simulink model "Examen3s"  (R2015b)
settings: Solver=VariableStepAuto  StartTime=0.0  StopTime=3  RelTol=1e-3
libraries: fl_lib x19, nesl_utility x8
settings Model: Creator=xmax1946  LastModifiedBy=xmax1946

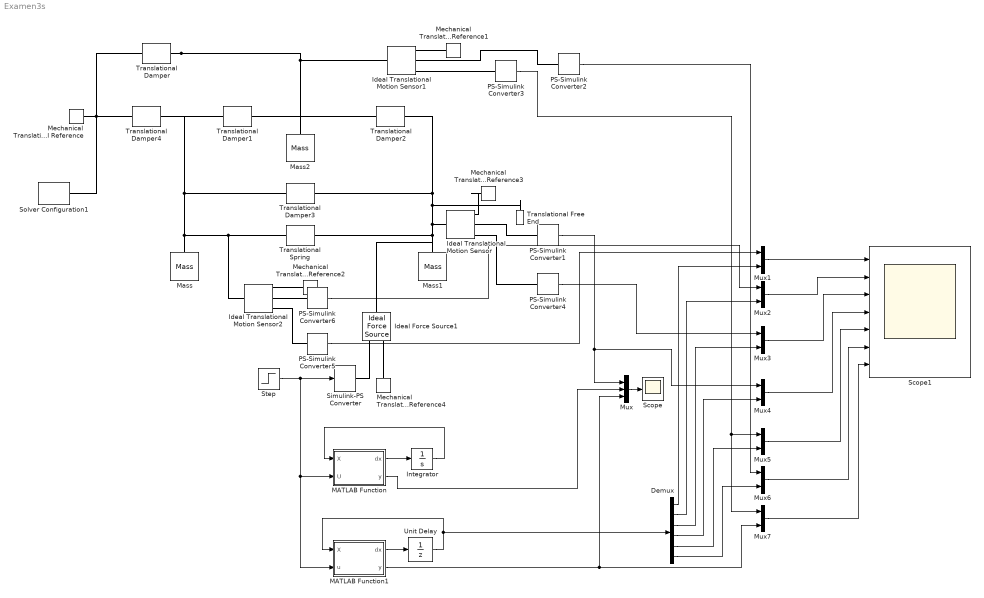
== system Examen3s ==
  Demux : Demux  Outputs=6
  Ideal Force Source1 : fl_lib/Mechanical/Mechanical Sources/Ideal Force Source
  Ideal Translational Motion Sensor : fl_lib/Mechanical/Mechanical Sensors/Ideal Translational Motion Sensor  offset=0 m
  Ideal Translational Motion Sensor1 : fl_lib/Mechanical/Mechanical Sensors/Ideal Translational Motion Sensor  offset=0 m
  Ideal Translational Motion Sensor2 : fl_lib/Mechanical/Mechanical Sensors/Ideal Translational Motion Sensor  offset=0 m
  Integrator : Integrator  InitialCondition=[0;0;0;0;0;0]
  MATLAB Function : MATLAB Function  TreatAsAtomicUnit=on
  MATLAB Function1 : MATLAB Function  TreatAsAtomicUnit=on
  Mass : fl_lib/Mechanical/Translational Elements/Mass  mass=2 kg  v_specify=off  v_priority=None  v=0 m/s  f_specify=off  f_priority=None  f=0 N
  Mass1 : fl_lib/Mechanical/Translational Elements/Mass  mass=1 kg  v_specify=off  v_priority=None  v=0 m/s  f_specify=off  f_priority=None  f=0 N
  Mass2 : fl_lib/Mechanical/Translational Elements/Mass  mass=1 kg  v_specify=off  v_priority=None  v=0 m/s  f_specify=off  f_priority=None  f=0 N
  Mechanical Translational Reference{,1..4} (5 alike) : fl_lib/Mechanical/Translational Elements/Mechanical Translational Reference
  Mux : Mux  Inputs=3
  Mux{1..7} (7 alike) : Mux  Inputs=2
  PS-Simulink Converter{1..6} (6 alike) : nesl_utility/PS-Simulink Converter  PhysicalDomain=network_engine_domain  SubClassName=ps_output  LeftPortType=input  RightPortType=output  PseudoPeriodic=off  Frequencies=[]  Unit=1  AffineConversion=off
  Scope : Scope
  Scope1 : Scope  NumInputPorts=7
  Simulink-PS Converter : nesl_utility/Simulink-PS Converter  PhysicalDomain=network_engine_domain  SubClassName=ps_input  LeftPortType=input  RightPortType=output  PseudoPeriodic=off  Frequencies=[]  NoiseDistribution=none  NoiseParameters=[]  Unit=1  AffineConversion=off  InputFiltering=off  SimscapeFilterOrder=1  InputFilterTimeConstant=0.001  UdotUserProvided=1
  Solver Configuration1 : nesl_utility/Solver Configuration  PhysicalDomain=network_engine_domain  SubClassName=solver  LeftPortType=input  RightPortType=generic  Accelerate=off  Tones=[]  Harmonics=[]  SimulateNoise=off  Profile=off  UseLocalSampling=off  EnableSwitchedLinearOptims=on  FrequencyDomain=off  UseCCode=off  RelTol=0.001  AbsTol=1e-06  MinStep=1e-09  ToWorkspace=off  RevertToSquareIcSolve=off  NumHomotopyIterations=100  PhasorMode=off  PhasorModeNumHarmonics=1  DoDC=off  ResidualTolerance=1e-09  UseLocalSolver=off  LocalSolverChoice=NE_BACKWARD_EULER_ADVANCER  LocalSolverSampleTime=0.001  DoFixedCost=off  MaxNonlinIter=3  MaxModeIter=2  LinearAlgebra=Sparse  DelaysMemoryBudget=1024  AutomaticFiltering=on  FilteringTimeConstant=0.001
  Step : Step  Time=0  SampleTime=0
  Translational Damper{,1..4} (5 alike) : fl_lib/Mechanical/Translational Elements/Translational Damper  D=1 N/(m/s)  v_specify=off  v_priority=None  v=0 m/s  f_specify=off  f_priority=None  f=0 N
  Translational Free End : fl_lib/Mechanical/Translational Elements/Translational Free End  v_specify=off  v_priority=None  v=0 m/s
  Translational Spring : fl_lib/Mechanical/Translational Elements/Translational Spring  spr_rate=2 N/m  v_specify=off  v_priority=None  v=0 m/s  f_specify=off  f_priority=None  f=0 N  x_specify=off  x_priority=None  x=0 m
  Unit Delay : UnitDelay  InitialCondition=[0;0;0;0;0;0]  SampleTime=.1
  wires:
  Step/1 -> MATLAB Function1/2(u), MATLAB Function/2(U), Simulink-PS Converter/1
  MATLAB Function/1(dx) -> Integrator/1
  MATLAB Function/2(y) -> Mux/2
  PS-Simulink Converter1/1 -> Mux4/1, Mux/1
  Mux/1 -> Scope/1
  Integrator/1 -> MATLAB Function/1(X)
  MATLAB Function1/2(y) -> Mux7/2, Mux/3
  MATLAB Function1/1(dx) -> Unit Delay/1
  Unit Delay/1 -> MATLAB Function1/1(X), Demux/1
  Mux1/1 -> Scope1/1
  Demux/1 -> Mux1/2
  Demux/2 -> Mux2/2
  Demux/3 -> Mux3/2
  Demux/4 -> Mux4/2
  Demux/5 -> Mux5/2
  Demux/6 -> Mux6/2
  PS-Simulink Converter4/1 -> Mux3/1
  PS-Simulink Converter3/1 -> Mux7/1, Mux5/1
  Mux2/1 -> Scope1/2
  Mux3/1 -> Scope1/3
  Mux4/1 -> Scope1/4
  Mux5/1 -> Scope1/5
  Mux6/1 -> Scope1/6
  Mux7/1 -> Scope1/7
  PS-Simulink Converter5/1 -> Mux1/1
  PS-Simulink Converter6/1 -> Mux2/1
  PS-Simulink Converter2/1 -> Mux6/1
  connections:
  Solver Configuration1/RConn1 -- Translational Damper4/LConn1 -- Translational Damper/LConn1 -- Mechanical Translational Reference/LConn1
  Translational Spring/LConn1 -- Ideal Translational Motion Sensor2/LConn1 -- Mass/LConn1 -- Translational Damper4/RConn1 -- Translational Damper1/LConn1 -- Translational Damper3/LConn1
  Translational Damper/RConn1 -- Ideal Translational Motion Sensor1/LConn1 -- Mass2/LConn1 -- Translational Damper2/LConn1 -- Translational Damper1/RConn1
  Translational Free End/LConn1 -- Translational Damper2/RConn1 -- Translational Damper3/RConn1 -- Ideal Translational Motion Sensor/LConn1 -- Translational Spring/RConn1 -- Mass1/LConn1 -- Ideal Force Source1/LConn1
  Ideal Translational Motion Sensor/RConn2 -- PS-Simulink Converter1/LConn1
  Mechanical Translational Reference2/LConn1 -- Ideal Translational Motion Sensor2/RConn1
  Mechanical Translational Reference1/LConn1 -- Ideal Translational Motion Sensor1/RConn1
  Mechanical Translational Reference4/LConn1 -- Ideal Force Source1/RConn2
  Mechanical Translational Reference3/LConn1 -- Ideal Translational Motion Sensor/RConn1
  Simulink-PS Converter/RConn1 -- Ideal Force Source1/RConn1
  PS-Simulink Converter6/LConn1 -- Ideal Translational Motion Sensor2/RConn2
  PS-Simulink Converter5/LConn1 -- Ideal Translational Motion Sensor2/RConn3
  PS-Simulink Converter4/LConn1 -- Ideal Translational Motion Sensor/RConn3
  PS-Simulink Converter2/LConn1 -- Ideal Translational Motion Sensor1/RConn2
  PS-Simulink Converter3/LConn1 -- Ideal Translational Motion Sensor1/RConn3

== matlab function Examen3s/MATLAB Function1 ==
  data: X input; dx output; u input; y output
function [dx,y] = fcn(X,u)

Av=[    0.99540503736190813541772738383712 - 2.3532845890485247962264745129938e-39i,  0.092863417010952603415329108868966 - 8.9876817216496555251003189708149e-39i,    0.0045949626380918645822726161628829 + 2.3016271224596547397239421456354e-39i, 0.0024483961633345975003348282607608 - 6.4846263527340942803335162399591e-39i,   0, 0.0022320933007049013847774850575472 - 4.0350221124417388579200282503283e-39i
 - 0.087966624684283408414659452347444 - 4.1268576085997300694800857922988e-39i,   0.86079040130951872917984603385198 + 2.8124620698384808540267622228462e-40i,     0.087966624684283408414659452347444 + 4.1268576085997300694800857922988e-39i,  0.048361972117603872674044999133391 + 6.5949365678457438801566322327557e-39i,   0,  0.042183824766696195053666927522602 + 1.7283727362859439738138954578664e-39i
   0.009197248478949766763265550191777 - 1.5956417457450973008559997917372e-39i, 0.0048967923266691950006696565215217 - 1.2969252705468188560667032479918e-38i,       0.99080275152105023323673444980822 + 2.066298663554802260101294694336e-39i,  0.090556781688449124125792403455011 - 1.5934893513038943818350609430973e-39i,   0, 0.0043151025578126469600365294022778 - 2.4042245908236605463886939308055e-39i
     0.1762167710502290532509151503885 + 9.6606637169324348723138656455673e-39i,  0.096723944235207745348089998266783 + 1.3189873135691487760313264465511e-38i,     - 0.1762167710502290532509151503885 - 9.6606637169324348723138656455673e-39i,   0.81645268686529922944552100056124 - 3.8456114016158819840774095700142e-39i,   0,   0.080059870178345780746017643508938 - 7.346839692639296924804603357639e-40i
  0.00014542244221413701015828177981097 - 2.496060086981651757948751472776e-39i, 0.0044641866014098027695549701150944 - 8.0700442248834777158400565006566e-39i, - 0.00014542244221413701015828177981097 + 2.5419778350606473637287802437612e-39i, 0.0043151025578126469600365294022778 - 2.4042245908236605463886939308055e-39i, 1.0,  0.086603404435480310291471499035757 - 3.8951164737635491215590030887326e-39i
  0.0041660185142154911505180886894612 + 3.4983584317684777153659419894383e-39i,  0.084367649533392390107333855045205 + 3.4567454725718879476277909157329e-39i,  - 0.0041660185142154911505180886894612 - 3.4983584317684777153659419894383e-39i,   0.080059870178345780746017643508938 - 7.346839692639296924804603357639e-40i,   0,   0.74673698255207661747039951735255 + 5.2674472962338435739925973340768e-39i];
A=real(Av);
B=[0.000082089719908973063781597233991388
   0.0024483961633345975003348282607608
   0.0046807139593838564454143723298798
     0.09055678168844912412579240345501
  0.00014923370716006084971981338719808
   0.0043151025578126469600365294022778];
C=[0,0,0,0,1,0];

dx=A*X+B*u;
y=C*X;

== matlab function Examen3s/MATLAB Function ==
  data: dx output; X input; y output; U input
function [dx,y] = fss(X,U)
m1=2;
m2=1;
m3=1;
v1=1;
v2=1;
v3=1;
v4=1;
v5=1;
k=2;
A=[0,1,0,0,0,0;
  -k/m1,(-v2-v4-v1)/m1,k/m1,v2/m1,0,v4/m1
  0,0,0,1,0,0 
  k/m2,v2/m2,-k/m2,(-v2-v5)/m2,0,v5/m2
  0,0,0,0,0,1
  0,v4/m3,0,v5/m3,0,(-v4-v3-v5)/m3
    ];
B=[0;0;0;1/m2;0;0];
C=[0,0,0,1,0,0];
u=U;
dx=A*X+B*u;
y=C*X;
